simulink model "model"  (R2019b)
settings: Solver=VariableStepAuto  StartTime=0.0  StopTime=1000  RelTol=1e-3
values from neighbouring files (symbols this model uses):
  c = temperature(1)    [Simulation.m]
  k = 21.39786113868873/duty    (= 21.3978611387)    [Simulation.m]
  ref = 37    [Simulation.m]
  T = 248.9986821828368    (= 248.998682183)    [Simulation.m]
libraries: simulink x1
settings Model: Creator=kacpe  LastModifiedBy=kacpe

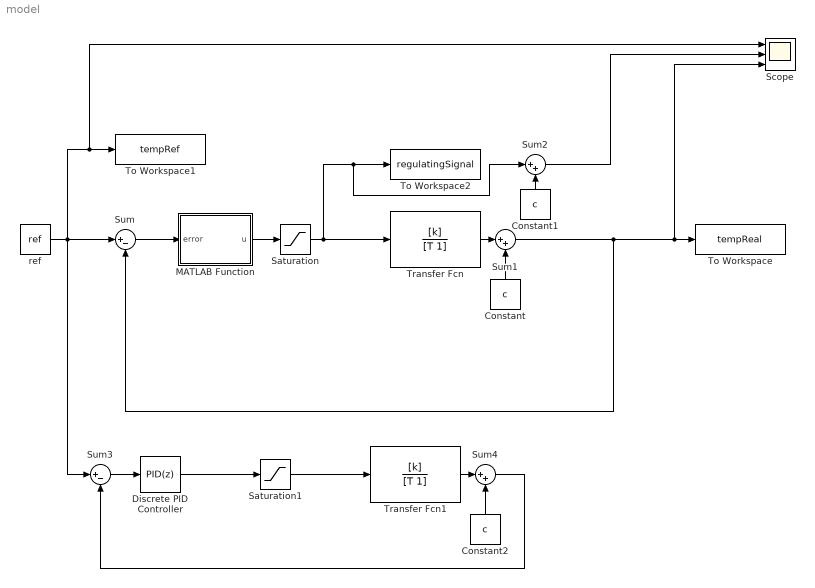
== system model ==
  Constant : Constant  Value=c
  Constant1 : Constant  Value=c
  Constant2 : Constant  Value=c
  Discrete PID Controller : simulink/Continuous/PID Controller  Controller=PID  Form=Parallel  TimeDomain=Discrete-time  SampleTime=1  IntegratorMethod=Trapezoidal  FilterMethod=Backward Euler  ControllerParametersSource=internal  P=0.0948667175981227  I=0.000482928713856668  D=1.50608802557373  UseFilter=on  N=0.0150390754087483  TunerSelectOption=Transfer Function Based (PID Tuner App)  InitialConditionSource=internal  InitialConditionForIntegrator=0  InitialConditionForFilter=0  DifferentiatorICPrevScaledInput=0  ExternalReset=none  TrackingMode=off  Kt=1  LimitOutput=on  UpperSaturationLimit=1  LowerSaturationLimit=0  LinearizeAsGain=off  AntiWindupMode=none  Kb=1  POutMin=[]  POutMax=[]  IOutMin=[]  IOutMax=[]  DOutMin=[]  DOutMax=[]  NOutMin=[]  NOutMax=[]  SumOutMin=[]  SumOutMax=[]  SaturationOutMin=[]  SaturationOutMax=[]  PParamMin=[]  PParamMax=[]  IParamMin=[]  IParamMax=[]  DParamMin=[]  DParamMax=[]  NParamMin=[]  NParamMax=[]  KbParamMin=[]  KbParamMax=[]  KtParamMin=[]  KtParamMax=[]  KbOutMin=[]  KbOutMax=[]  KtOutMin=[]  KtOutMax=[]  IntegratorOutMin=[]  IntegratorOutMax=[]  FilterOutMin=[]  FilterOutMax=[]  SumI1OutMin=[]  SumI1OutMax=[]  SumI2OutMin=[]  SumI2OutMax=[]  SumI3OutMin=[]  SumI3OutMax=[]  SumI4OutMin=[]  SumI4OutMax=[]  SumDOutMin=[]  SumDOutMax=[]  DifferentiatorOutMin=[]  DifferentiatorOutMax=[]  FilterDiffOutCoefMin=[]  FilterDiffOutCoefMax=[]  ReciprocalOutMin=[]  ReciprocalOutMax=[]  SumDenOutMin=[]  SumDenOutMax=[]  SumNumOutMin=[]  SumNumOutMax=[]  DivideOutMin=[]  DivideOutMax=[]  IntegratorContinuousStateAttributes=''  IntegratorStateMustResolveToSignalObject=off  IntegratorRTWStateStorageClass=Auto  FilterContinuousStateAttributes=''  FilterStateMustResolveToSignalObject=off  FilterRTWStateStorageClass=Auto  ParallelPVariant=InternalParameters  IdealPVariant=Disabled  IVariant=InternalParameters  DVariant=InternalParameters  IntegratorVariant=Discrete  SatVariant=Enabled  AWVariant=Passthrough  PCopyVariant=Disabled  TRVariant=Disabled  FdbkBlocksVariant=Forward  IdealPFdbkVariant=Disabled  SatFdbkVariant=Disabled  DerivativeFilterVariant=BackwardEulerFilter  NVariant=InternalParameters  NCopyVariant=InternalParameters  FilterICVariant=InternalICsFilter  IntegratorICVariant=InternalICs  ExternalResetVariant=Disabled  TRSumVariant=Passthrough  SumFdbkVariant=Disabled  SumVariant=Sum_PID
  MATLAB Function : MATLAB Function  TreatAsAtomicUnit=on
  Saturation : Saturate  UpperLimit=1  LowerLimit=0
  Saturation1 : Saturate  UpperLimit=1  LowerLimit=0
  Scope : Scope  NumInputPorts=3
  Sum : Sum  Inputs=|+-
  Sum1 : Sum  Inputs=|++
  Sum2 : Sum  Inputs=|++
  Sum3 : Sum  Inputs=|+-
  Sum4 : Sum  Inputs=|++
  To Workspace : ToWorkspace  VariableName=tempReal  SampleTime=-1
  To Workspace1 : ToWorkspace  VariableName=tempRef  SampleTime=-1
  To Workspace2 : ToWorkspace  VariableName=regulatingSignal  SampleTime=-1
  Transfer Fcn : TransferFcn  Numerator=[k]  Denominator=[T 1]
  Transfer Fcn1 : TransferFcn  Numerator=[k]  Denominator=[T 1]
  ref : Constant  Value=ref
  wires:
  Transfer Fcn/1 -> Sum1/1
  Sum1/1 -> Sum/2, Scope/3, To Workspace/1
  Constant/1 -> Sum1/2
  Sum/1 -> MATLAB Function/1(error)
  Sum2/1 -> Scope/2
  Constant1/1 -> Sum2/2
  MATLAB Function/1(u) -> Saturation/1
  Saturation/1 -> Transfer Fcn/1, Sum2/1, To Workspace2/1
  Sum4/1 -> Sum3/2
  ref/1 -> Sum3/1, Sum/1, Scope/1, To Workspace1/1
  Discrete PID Controller/1 -> Saturation1/1
  Sum3/1 -> Discrete PID Controller/1
  Constant2/1 -> Sum4/2
  Saturation1/1 -> Transfer Fcn1/1
  Transfer Fcn1/1 -> Sum4/1

== matlab function model/MATLAB Function ==
  settings: updateMethod=DISCRETE  sampleTime=1
  data: error input; u output
function u = PID(error)
%@author Dominik Łuczak

%Declare static value
persistent previous_error;
if isempty(previous_error)
    previous_error = 0;
end

persistent previous_integral;
if isempty(previous_integral)
    previous_integral = 0;
end

%Constant values
dt = 1;
Kp = 0.0948667175981227
Ki = 0.000482928713856668;
Kd = 1.50608802557373

%proportional part 
P = Kp*error;

%integral part
integral = previous_integral + (error+previous_error) ; %numerical integrator without anti-windup
previous_integral = integral;
I = Ki*integral*(dt/2);

%derivative part
derivative = (error - previous_error)/dt; %numerical derivative without filter
previous_error = error;
D = Kd*derivative;


%sum of all parts
u = P  + I + D; %without saturation
end
